simulink model "HCSPWareHouseModel"  (R2017b)
settings: Solver=VariableStepAuto  StartTime=0.0  StopTime=10.0  RelTol=1e-3
settings Model: Creator=georgimarkov  LastModifiedBy=georgimarkov

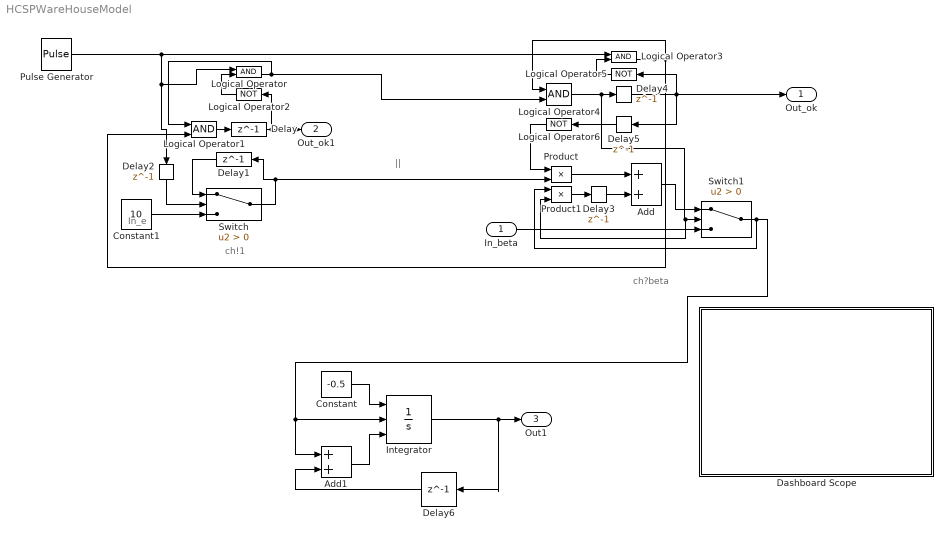
== system HCSPWareHouseModel ==
  note: ||
  note: ch?beta
  note: ch!1
  note: In_e
  "In_beta " : Inport
  Add : Sum
  Add1 : Sum
  Constant : Constant  Value=-0.5
  Constant1 : Constant  Value=10
  Dashboard Scope : Subsystem  DialogController=hmiCreateDDGDialog  IsWebBlock=on  mask(MWDashboardBlock){webBlockId=8eaaedce-aa2d-43e7-91f4-63c89c4a16ed, webBlockType=sdiscope, ShowInitialText=on, HMISrcModelName=untitled}
      mask prompts: webBlockId "WebBlock Id"; webBlockType "WebBlock Type"; HMISrcModelName "Source Model"
      mask help: SimulinkHMI:dialogs:HMIScopeDialogDesc
      mask Help: helpview([docroot '/mapfiles/simulink.map'], 'hmi_scope')
      mask Display:
      | if strcmp(get_param(bdroot(gcb),'BlockDiagramType'), 'library')
      |     image([(matlabroot) '/toolbox/simulink/hmi/icons/DashboardScope.png']);
      | end
  Delay{,1..6} (7 alike) : Delay  DelayLength=1  InitialCondition=0
  Integrator : Integrator  ExternalReset=rising  InitialConditionSource=external  ZeroCross=off
  Logical Operator{,1,3..4} (4 alike) : Logic  AllPortsSameDT=off  OutDataTypeStr=fixdt(1,16)
  Logical Operator2 : Logic  Operator=NOT  AllPortsSameDT=off  OutDataTypeStr=boolean
  Logical Operator5 : Logic  Operator=NOT  AllPortsSameDT=off  OutDataTypeStr=fixdt(1,16)
  Logical Operator6 : Logic  Operator=NOT  AllPortsSameDT=off  OutDataTypeStr=fixdt(1,16)
  Product : Product
  Product1 : Product
  Pulse Generator : DiscretePulseGenerator  PulseType=Time based  Period=100  PhaseDelay=5
  Switch : Switch  Criteria=u2 > Threshold
  Switch1 : Switch  Criteria=u2 > Threshold
  Out_ok : Outport
  Out_ok1 : Outport  Port=2
  Out1 : Outport  Port=3
  wires:
  Logical Operator/1 -> Logical Operator4/2, Logical Operator1/1
  Logical Operator6/1 -> Product/1
  Delay5/1 -> Logical Operator6/1
  Product/1 -> Add/1
  Delay3/1 -> Add/2
  Pulse Generator/1 -> Logical Operator3/1, Logical Operator/1, Delay2/1
  "In_beta "/1 -> Switch1/3
  Add/1 -> Switch1/1
  Delay4/1 -> Delay5/1, Logical Operator5/1, Out_ok/1
  Product1/1 -> Delay3/1
  Logical Operator5/1 -> Logical Operator3/2
  Logical Operator4/1 -> Product1/2, Switch1/2, Delay4/1
  Switch1/1 -> Add1/1, Integrator/2, Product1/1
  Switch/1 -> Product/2, Delay1/1
  Constant/1 -> Integrator/1
  Delay/1 -> Out_ok1/1, Logical Operator2/1
  Delay2/1 -> Switch/2
  Logical Operator3/1 -> Logical Operator1/2, Logical Operator4/1
  Logical Operator1/1 -> Delay/1
  Logical Operator2/1 -> Logical Operator/2
  Delay1/1 -> Switch/1
  Constant1/1 -> Switch/3
  Integrator/1 -> Delay6/1, Out1/1
  Add1/1 -> Integrator/3
  Delay6/1 -> Add1/2

== system HCSPWareHouseModel/Dashboard Scope ==
